simulink model "controller_testing_2WD_NO_REGEN"  (R2023b)
settings: Solver=VariableStepAuto  StartTime=0.0  StopTime=20  RelTol=1e-3
libraries: simulink x1
settings Model: Creator=Inver  LastModifiedBy=TAK
settings DataIOCC: ExternalInput=x2023_5_11_controller_testing_RA.getElement('left_temp_motor'),x2023_5_11_controller_testing_RA.getElement('right_temp_motor'),x2023_5_11_controller_testing_RA.getElement('left_temp_controller'),x2023_5_11_controller_testing_RA.getElement('right_temp_controller'),x2023_5_11_controller_testing_RA.getElement('left_wheel_omega'),x2023_5_11_controller_testing_RA.getElement('right_wheel_omega'),x2023_5_11_controller_testing_RA.getElement('pack_current_limit'),x2023_5_11_controller_testing_RA.getElement('pack_current'),x2023_5_11_controller_testing_RA.getElement('pack_voltage'),x2023_5_11_controller_testing_RA.getElement('gps_vel_n'),x2023_5_11_controller_testing_RA.getElement('gps_vel_e'),x2023_5_11_controller_testing_RA.getElement('gps_vel_d'),x2023_5_11_controller_testing_RA.getElement('imu_gyro_x'),x2023_5_11_controller_testing_RA.getElement('imu_gyro_y'),x2023_5_11_controller_testing_RA.getElement('imu_gyro_z'),x2023_5_11_controller_testing_RA.getElement('imu_accel_x'),x2023_5_11_controller_testing_RA.getElement('imu_accel_y'),x2023_5_11_controller_testing_RA.getElement('imu_accel_z'),x2023_5_11_controller_testing_RA.getElement('throttle'),x2023_5_11_controller_testing_RA.getElement('steering_angle')  LoadExternalInput=on
settings OptimizationCC: DefaultParameterBehavior=Inlined  UseDivisionForNetSlopeComputation=on  GainParamInheritBuiltInType=on  UseFloatMulNetSlope=on  InlineInvariantSignals=on  PassReuseOutputArgsAs=Individual arguments  ZeroExternalMemoryAtStartup=off  ZeroInternalMemoryAtStartup=off  NoFixptDivByZeroProtection=on  EfficientFloat2IntCast=on  LifeSpan=1  OptimizeBlockOrder=speed  OptimizationPriority=Speed  MultiThreadedLoops=on  EfficientTunableParamExpr=on
settings DebuggingCC: ParameterTunabilityLossMsg=error
settings HardwareCC: ProdBitPerPointer=32  ProdBitPerSizeT=32  ProdBitPerPtrDiffT=32  ProdLargestAtomicInteger=Long  ProdLargestAtomicFloat=Double  ProdWordSize=32  ProdLongLongMode=on  ProdHWDeviceType=ARM Compatible->ARM Cortex-M
settings SFSimCC: SimCustomHeaderCode="#include \"simplex.h\""  SimUserSources=simplex.c  MATLABDynamicMemAlloc=off
settings RTWCC: Description=Embedded Coder  SystemTargetFile=ert.tlc  GenCodeOnly=on  PackageGeneratedCodeAndArtifacts=on  TemplateMakefile=ert_default_tmf  Toolchain=GNU Tools for ARM Embedded Processors  BuildConfiguration=Faster Runs  CodeExecutionProfiling=on  CodeProfilingInstrumentation=detailed
settings CodeAppCC: ForceParamTrailComments=on  IgnoreCustomStorageClasses=off  OperatorAnnotations=on  SimulinkDataObjDesc=on  SFDataObjDesc=on  CustomSymbolStrGlobalVar=rt$N$M  CustomSymbolStrType=$N$M  CustomSymbolStrFcn=$N$M$F  CustomSymbolStrMacro=$N$M  InsertBlockDesc=on
settings ERTTargetCC: TargetLangStandard=C99 (ISO)  GenerateSampleERTMain=on  IncludeMdlTerminateFcn=off  CombineSignalStateStructs=on  CodeInterfacePackaging=Reusable function  SupportComplex=off  SupportNonInlinedSFcns=on  InlinedParameterPlacement=NonHierarchical  RootIOFormat=Structure reference  ERTCustomFileTemplate=example_file_process.tlc  GlobalDataDefinition=InSeparateSourceFile  DataDefinitionFile=data.c  GlobalDataReference=InSeparateHeaderFile  ERTFilePackagingFormat=CompactWithDataFile  DataReferenceFile=data.h

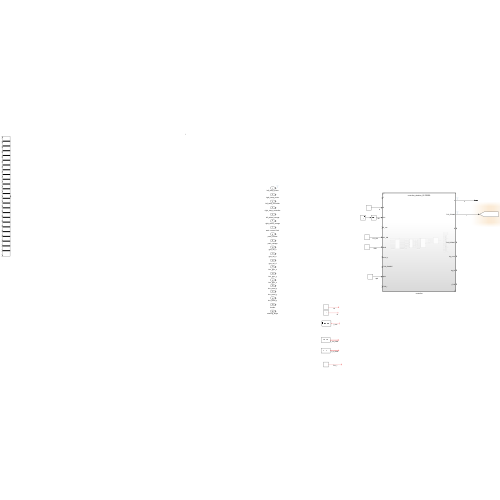
[thumbnail: Simulink's stored preview of the top-level diagram]
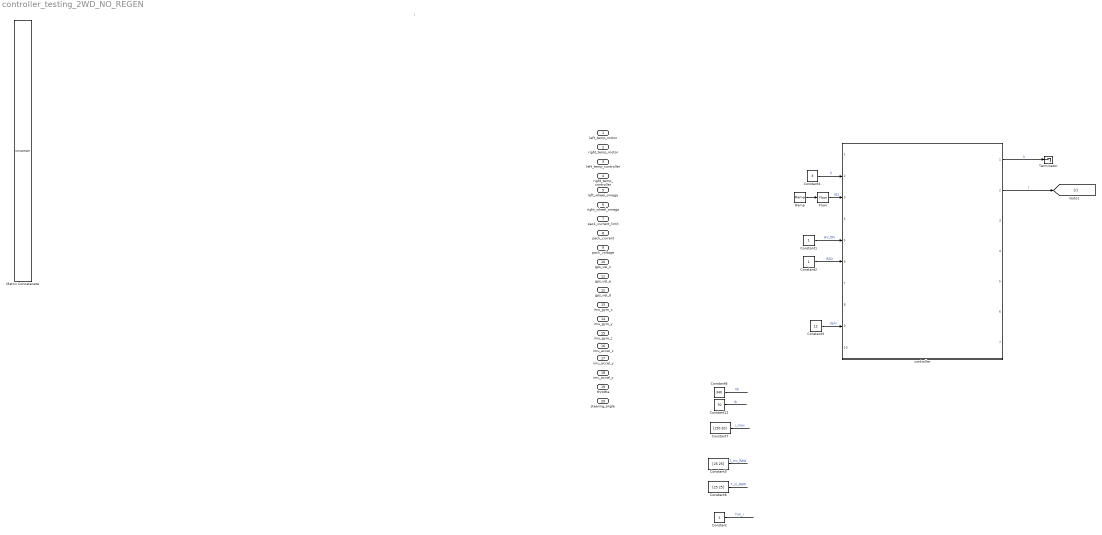
== system controller_testing_2WD_NO_REGEN ==
  note: l
  left_temp_motor : Inport
  right_temp_motor : Inport  Port=2
  left_temp_controller : Inport  Port=3
  right_temp_controller : Inport  Port=4
  left_wheel_omega : Inport  Port=5
  right_wheel_omega : Inport  Port=6
  pack_current_limit : Inport  Port=7
  pack_current : Inport  Port=8
  pack_voltage : Inport  Port=9
  gps_vel_n : Inport  Port=10
  gps_vel_e : Inport  Port=11
  gps_vel_d : Inport  Port=12
  imu_gyro_x : Inport  Port=13
  imu_gyro_y : Inport  Port=14
  imu_gyro_z : Inport  Port=15
  imu_accel_x : Inport  Port=16
  imu_accel_y : Inport  Port=17
  imu_accel_z : Inport  Port=18
  throttle : Inport  Port=19
  steering_angle : Inport  Port=20
  Constant : Constant
  Constant1 : Constant
  Constant12 : Constant  Value=70
  Constant2 : Constant
  Constant3 : Constant  Value=12
  Constant4 : Constant  Value=3
  Constant5 : Constant  Value=[25 25]
  Constant6 : Constant  Value=[25 25]
  Constant7 : Constant  Value=[150 20]
  Constant8 : Constant  Value=340
  Floor : Rounding
  Matrix Concatenate : Concatenate  NumInputs=25  ConcatenateDimension=2
  Ramp : simulink/Sources/Ramp  slope=50  start=0  InitialOutput=zeros(1,10)
  Terminator : Terminator
  controller : Subsystem  TreatAsAtomicUnit=on  SystemSampleTime=0.02  ReferencedSubsystem=controller_skeleton_FILTERED
  wires:
  Constant/1 -> ?  "TVV_I"
  Constant3/1 -> controller/9  "dphi"
  Constant2/1 -> controller/6  "R2D"
  Constant1/1 -> controller/5  "HV_ON"
  Constant4/1 -> controller/2  "S"
  Constant5/1 -> ?  "T_mc_RAW"
  Constant6/1 -> ?  "T_m_RAW"
  Constant7/1 -> ?  "i_max"
  Ramp/1 -> Floor/1
  Floor/1 -> controller/3  "ID1"
  Constant8/1 -> ?  "Vb"
  controller/1 -> Terminator/1  "k"
  Constant12/1 -> ?  "Ib"
  controller/2 -> [r]  "r"
